simulink model "controle_autonomo"  (R2023a)
settings: configuration reference "Configuration" (kept outside this file)
libraries: drivingvehiclecontroller x1
settings Model: DataDictionary=controle_autonomo_dict.sldd  Creator=thailon  LastModifiedBy=thailon
settings ConfigSetRef: SourceName=Configuration

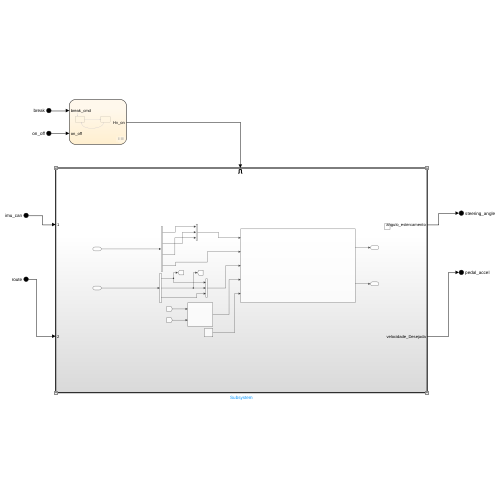
[thumbnail: Simulink's stored preview of the top-level diagram]
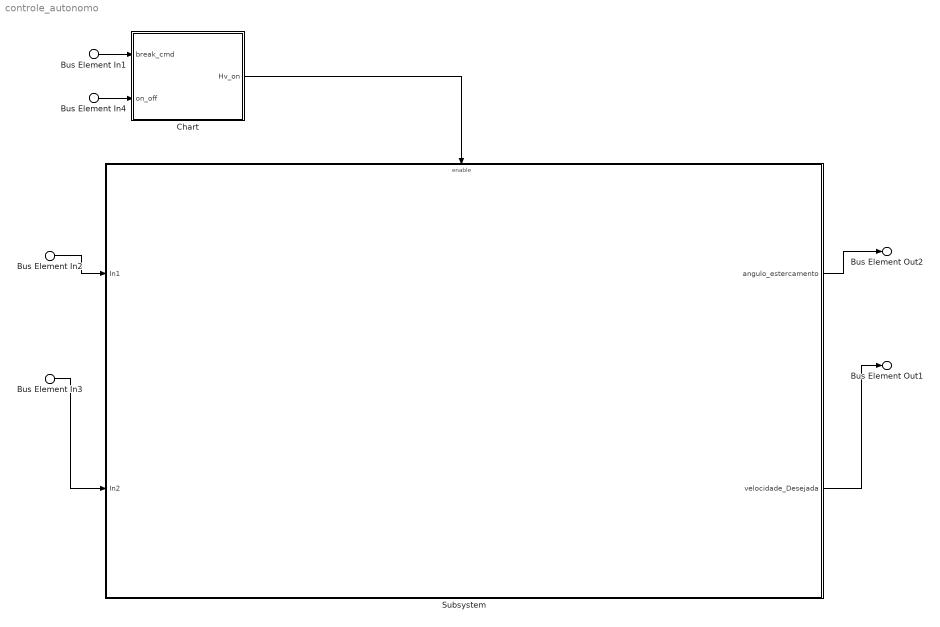
== system controle_autonomo ==
  Bus Element In1 : Inport  PortName=break
  Bus Element In2 : Inport  Port=2  PortName=imu_can
  Bus Element In3 : Inport  Port=3  PortName=route
  Bus Element In4 : Inport  Port=4  PortName=on_off
  Chart : Stateflow chart  TreatAsAtomicUnit=on
  Subsystem : Subsystem
  Bus Element Out1 : Outport  PortName=pedal_accel
  Bus Element Out2 : Outport  Port=2  PortName=steering_angle
  wires:
  Bus Element In1/1 -> Chart/1(break_cmd)
  Bus Element In4/1 -> Chart/2(on_off)
  Bus Element In2/1 -> Subsystem/1(In1)
  Bus Element In3/1 -> Subsystem/2(In2)
  Subsystem/1(angulo_estercamento) -> Bus Element Out2/1
  Subsystem/2(velocidade_Desejada) -> Bus Element Out1/1
  Chart/1(Hv_on) -> Subsystem/Enable

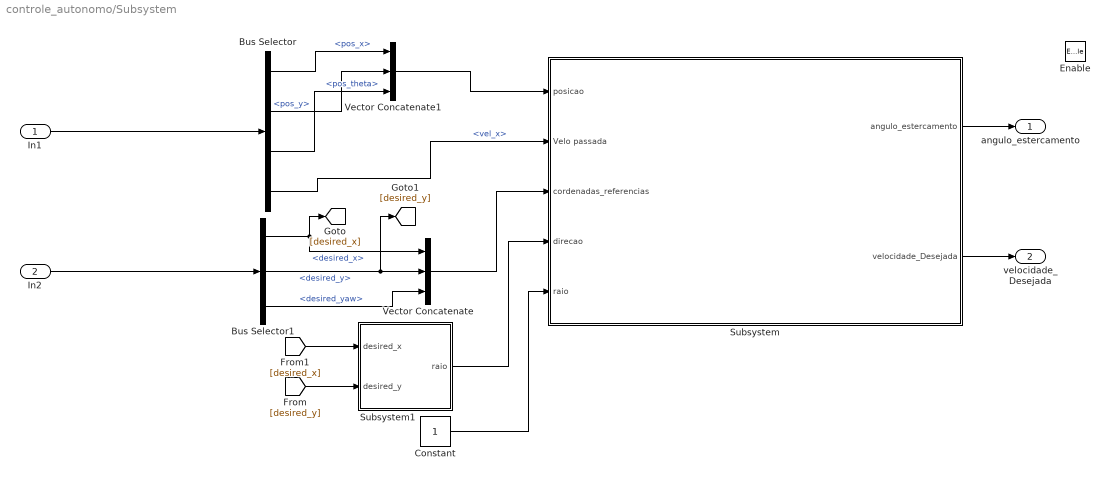
== system controle_autonomo/Subsystem ==
  In1 : Inport
  In2 : Inport  Port=2
  Enable : EnablePort
  Bus Selector : BusSelector  OutputSignals=pos_x,pos_y,pos_theta,vel_x
  Bus Selector1 : BusSelector  OutputSignals=desired_x,desired_y,desired_yaw
  Constant : Constant
  Subsystem : Subsystem
  Subsystem1 : Subsystem
  Vector Concatenate : Concatenate  NumInputs=3
  Vector Concatenate1 : Concatenate  NumInputs=3
  angulo_estercamento : Outport
  velocidade_Desejada : Outport  Port=2
  wires:
  Subsystem1/1(raio) -> Subsystem/4(direcao)
  [desired_y] -> Subsystem1/2(desired_y)
  Bus Selector/4 -> Subsystem/2(Velo passada)  "<vel_x>"
  Subsystem/1(angulo_estercamento) -> angulo_estercamento/1
  Bus Selector/1 -> Vector Concatenate1/1  "<pos_x>"
  Bus Selector1/1 -> Vector Concatenate/1, [desired_x]  "<desired_x>"
  Bus Selector/2 -> Vector Concatenate1/2  "<pos_y>"
  [desired_x] -> Subsystem1/1(desired_x)
  In1/1 -> Bus Selector/1
  Bus Selector1/2 -> Vector Concatenate/2, [desired_y]  "<desired_y>"
  Vector Concatenate/1 -> Subsystem/3(cordenadas_referencias)
  Bus Selector1/3 -> Vector Concatenate/3  "<desired_yaw>"
  In2/1 -> Bus Selector1/1
  Constant/1 -> Subsystem/5(raio)
  Bus Selector/3 -> Vector Concatenate1/3  "<pos_theta>"
  Subsystem/2(velocidade_Desejada) -> velocidade_Desejada/1
  Vector Concatenate1/1 -> Subsystem/1(posicao)

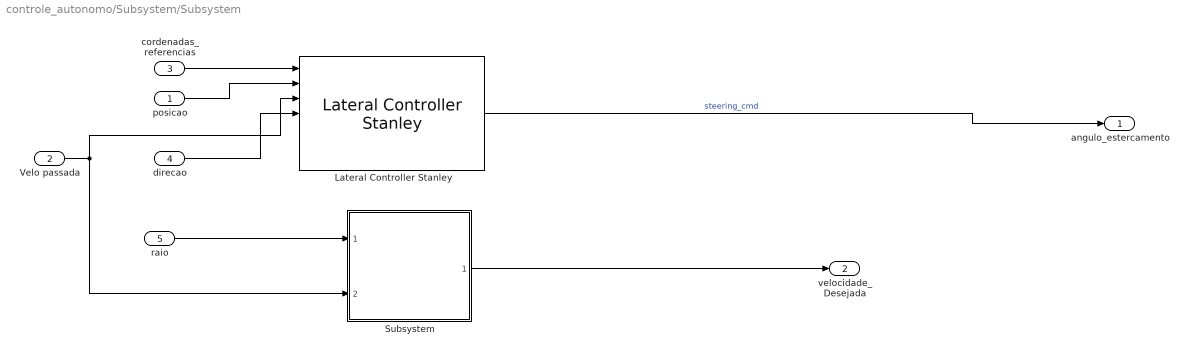
== system controle_autonomo/Subsystem/Subsystem ==
  posicao : Inport
  Velo passada : Inport  Port=2
  cordenadas_referencias : Inport  Port=3
  direcao : Inport  Port=4
  raio : Inport  Port=5
  Lateral Controller Stanley : drivingvehiclecontroller/Lateral Controller Stanley  ModelType=Dynamic bicycle model  PositionGainF=stanley_kpfw  PositionGainR=stanley_kprv  YawRateGain=1  DelayGain=0.2  VehicleMass=230  Lf=1.4  Lr=1.6  TireStiffness=12e3  Wheelbase=wheelbase  MaxSteeringAngle=max_steering_angle
  Subsystem : Subsystem  ReferencedSubsystem=pid_longitudinal
  angulo_estercamento : Outport
  velocidade_Desejada : Outport  Port=2
  wires:
  direcao/1 -> Lateral Controller Stanley/4
  posicao/1 -> Lateral Controller Stanley/2
  Lateral Controller Stanley/1 -> angulo_estercamento/1  "steering_cmd"
  cordenadas_referencias/1 -> Lateral Controller Stanley/1
  Subsystem/1 -> velocidade_Desejada/1
  Velo passada/1 -> Subsystem/2, Lateral Controller Stanley/3
  raio/1 -> Subsystem/1

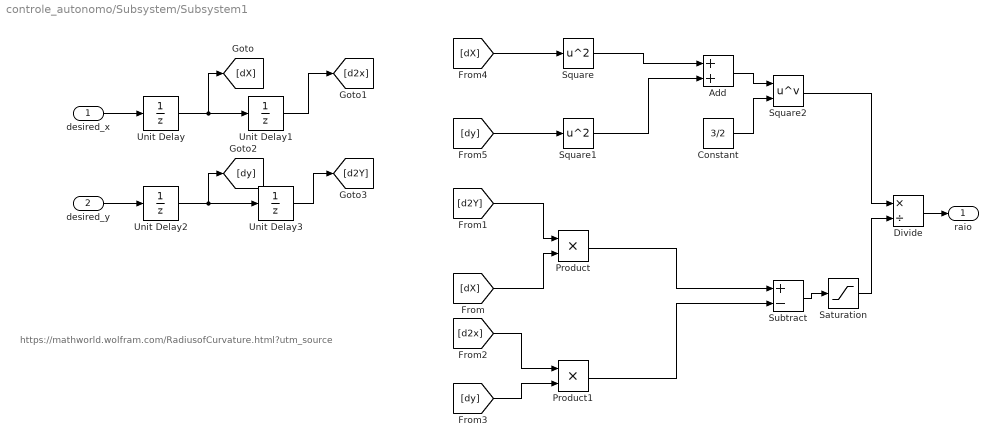
== system controle_autonomo/Subsystem/Subsystem1 ==
  note: https://mathworld.wolfram.com/RadiusofCurvature.html?utm_source
  desired_x : Inport
  desired_y : Inport  Port=2
  Add : Sum
  Constant : Constant  Value=3/2
  Divide : Product  Inputs=*/
  Product : Product
  Product1 : Product
  Saturation : Saturate  UpperLimit=10000  LowerLimit=0.00001
  Square : Math  Operator=square
  Square1 : Math  Operator=square
  Square2 : Math  Operator=pow
  Subtract : Sum  Inputs=+-
  Unit Delay{,1..3} (4 alike) : UnitDelay  SampleTime=-1  HasFrameUpgradeWarning=on
  raio : Outport
  wires:
  [dX] -> Square/1
  [d2x] -> Product1/1
  desired_x/1 -> Unit Delay/1
  [dy] -> Product1/2
  Product/1 -> Subtract/1
  Unit Delay1/1 -> [d2x]
  Add/1 -> Square2/1
  Unit Delay/1 -> [dX], Unit Delay1/1
  Square1/1 -> Add/2
  [d2Y] -> Product/1
  [dy] -> Square1/1
  Product1/1 -> Subtract/2
  [dX] -> Product/2
  desired_y/1 -> Unit Delay2/1
  Unit Delay2/1 -> [dy], Unit Delay3/1
  Constant/1 -> Square2/2
  Unit Delay3/1 -> [d2Y]
  Divide/1 -> raio/1
  Square2/1 -> Divide/1
  Subtract/1 -> Saturation/1
  Saturation/1 -> Divide/2
  Square/1 -> Add/1

== stateflow chart controle_autonomo/Chart ==
  state Idle
  state HV
    entry:
    Hv_on = 1;
  (default) -> Idle
  Idle -> HV : [on_off==true]
  HV -> Idle : [(on_off == false) || (break_cmd == true) ]
  data: break_cmd input; on_off input; Hv_on output
